simulink model "basic"  (Simulink 5.0)
settings: Solver=ode45  StartTime=t_init  StopTime=t_final  RelTol=1e-3
undefined symbols (not defined in the file or in its folder): den, gamma, num, Rc, Sc, st, Tc, Ts
settings Model: Creator=kannan  LastModifiedBy=kannan  ExtModeAutoUpdateStatusClock=off

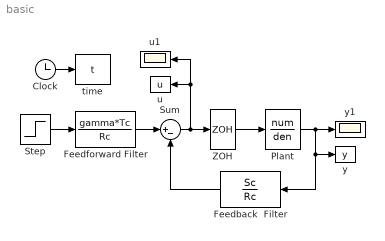
== system basic ==
  Clock : Clock
      settings: Decimation=10
  Feedback  Filter : DiscreteFilter  Orientation=left  Numerator=Sc  Denominator=Rc  SampleTime=Ts
  Feedforward Filter : DiscreteFilter  Numerator=gamma*Tc  Denominator=Rc  SampleTime=Ts
  Plant : TransferFcn  Numerator=num  Denominator=den
  Step : Step  Time=0  After=st  SampleTime=Ts
  Sum : Sum  Inputs=|+-  SaturateOnIntegerOverflow=on
  ZOH : ZeroOrderHold  SampleTime=Ts
  time : ToWorkspace  VariableName=t  SampleTime=Ts  SaveFormat=Array
  u : ToWorkspace  VariableName=u  SampleTime=Ts  SaveFormat=Array
  u1 : Scope
      settings: YMin=-6e+164  YMax=1.02293e+149
  y : ToWorkspace  VariableName=y  SampleTime=Ts  SaveFormat=Array
  y1 : Scope
      settings: YMin=-6e+164  YMax=1.02293e+149
  wires:
  Feedforward Filter/1 -> Sum/1
  Feedback  Filter/1 -> Sum/2
  Clock/1 -> time/1
  Sum/1 -> ZOH/1, u1/1, u/1
  ZOH/1 -> Plant/1
  Step/1 -> Feedforward Filter/1
  Plant/1 -> y1/1, Feedback  Filter/1, y/1
